simulink model "guid_stab_loop_no_rot_simtemp"  (R2021a)
settings: Solver=VariableStepAuto  StartTime=0.0  StopTime=20  RelTol=1e-3
settings Model: Creator=AutomZ2-RG02A02  LastModifiedBy=AutomZ2-RG02A02

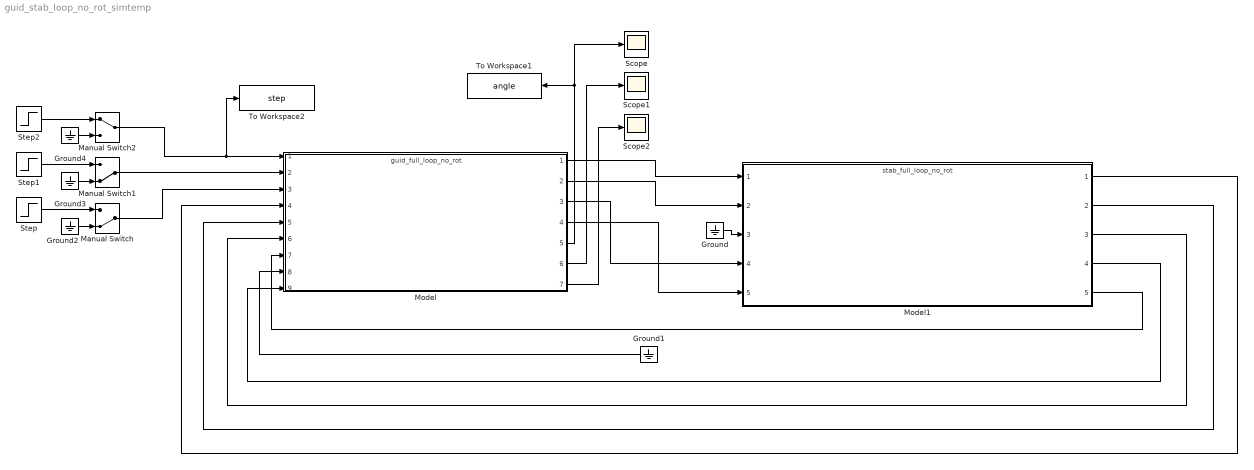
== system guid_stab_loop_no_rot_simtemp ==
  Ground{,1..4} (5 alike) : Ground
  Manual Switch : ManualSwitch  CurrentSetting=0
  Manual Switch1 : ManualSwitch  CurrentSetting=0
  Manual Switch2 : ManualSwitch
  Model : ModelReference  ModelNameDialog=guid_full_loop_no_rot.slx  SimulationMode=Normal  ModelReferenceVersion=73
  Model1 : ModelReference  ModelNameDialog=stab_full_loop_no_rot.slx  SimulationMode=Normal  ModelReferenceVersion=63
  Scope : Scope
  Scope1 : Scope
  Scope2 : Scope
  Step : Step  SampleTime=0
  Step1 : Step  SampleTime=0
  Step2 : Step  SampleTime=0
  To Workspace1 : ToWorkspace  VariableName=angle  SaveFormat=Structure With Time  SampleTime=0.002
  To Workspace2 : ToWorkspace  VariableName=step  SaveFormat=Structure With Time  SampleTime=0.002
  wires:
  Model/1 -> Model1/1
  Model/2 -> Model1/2
  Model/3 -> Model1/4
  Model/4 -> Model1/5
  Ground/1 -> Model1/3
  Manual Switch2/1 -> To Workspace2/1, Model/1
  Manual Switch1/1 -> Model/2
  Model1/1 -> Model/4
  Model1/2 -> Model/5
  Model1/3 -> Model/6
  Model1/5 -> Model/7
  Ground1/1 -> Model/8
  Model1/4 -> Model/9
  Step/1 -> Manual Switch/1
  Manual Switch/1 -> Model/3
  Ground2/1 -> Manual Switch/2
  Ground3/1 -> Manual Switch1/2
  Step1/1 -> Manual Switch1/1
  Ground4/1 -> Manual Switch2/2
  Model/5 -> Scope/1, To Workspace1/1
  Model/6 -> Scope1/1
  Model/7 -> Scope2/1
  Step2/1 -> Manual Switch2/1
